simulink model "clase08122020"  (R2020b)
settings: Solver=VariableStepDiscrete  StartTime=0.0  StopTime=inf  MaxStep=1e-6/2  RelTol=1e-3
libraries: hdlsllib x4
settings Model: Creator=fer-1  LastModifiedBy=fer-1

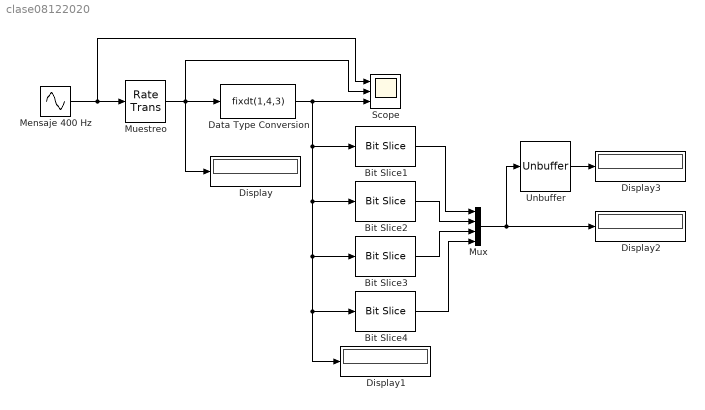
== system clase08122020 ==
  Bit Slice1 : hdlsllib/Logic and Bit Operations/Bit Slice  lidx=3  ridx=3
      settings: SourceProductBaseCode=SL
  Bit Slice2 : hdlsllib/Logic and Bit Operations/Bit Slice  lidx=2  ridx=2
      settings: SourceProductBaseCode=SL
  Bit Slice3 : hdlsllib/Logic and Bit Operations/Bit Slice  lidx=1  ridx=1
      settings: SourceProductBaseCode=SL
  Bit Slice4 : hdlsllib/Logic and Bit Operations/Bit Slice  lidx=0  ridx=0
      settings: SourceProductBaseCode=SL
  Data Type Conversion : DataTypeConversion  OutDataTypeStr=fixdt(1,4,3)
  Display{,1..3} (4 alike) : Display
  Mensaje 400 Hz : Sin  Frequency=400*pi  SampleTime=0
  Muestreo : RateTransition  OutPortSampleTime=1/4000
  Mux : Mux
  Scope : Scope  NumInputPorts=3
  Unbuffer : Unbuffer
  wires:
  Mensaje 400 Hz/1 -> Scope/1, Muestreo/1
  Data Type Conversion/1 -> Bit Slice2/1, Bit Slice3/1, Display1/1, Bit Slice4/1, Bit Slice1/1, Scope/3
  Muestreo/1 -> Display/1, Scope/2, Data Type Conversion/1
  Bit Slice1/1 -> Mux/1
  Bit Slice2/1 -> Mux/2
  Bit Slice3/1 -> Mux/3
  Bit Slice4/1 -> Mux/4
  Mux/1 -> Unbuffer/1, Display2/1
  Unbuffer/1 -> Display3/1
